simulink model "enfas"  (R2020b)
settings: Solver=VariableStepAuto  StartTime=0.0  StopTime=stop_time  RelTol=tolerance
model workspace (MAT data in the model file):
  R = 40
  a = 220
  freq = 314.16
values from neighbouring files (symbols this model uses):
  amplitude = 220    [lab1.m]
  L = 95 * 10^-3    (= 0.095)    [lab1.m]
settings Model: Creator=axelfroborg  LastModifiedBy=axelfroborg

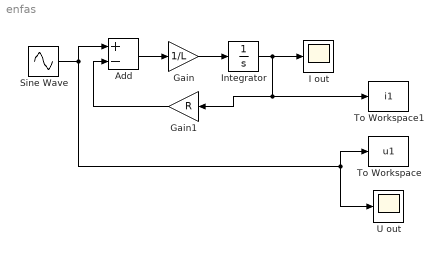
== system enfas ==
  Add : Sum  Inputs=+-
  Gain : Gain  Gain=1/L
  Gain1 : Gain  Gain=R
  I out : Scope
  Integrator : Integrator
  Sine Wave : Sin  Amplitude=amplitude  Frequency=freq  SampleTime=0
  To Workspace : ToWorkspace  VariableName=u1  SampleTime=-1
  To Workspace1 : ToWorkspace  VariableName=i1  SampleTime=-1
  U out : Scope
  wires:
  Integrator/1 -> Gain1/1, To Workspace1/1, I out/1
  Add/1 -> Gain/1
  Gain/1 -> Integrator/1
  Gain1/1 -> Add/2
  Sine Wave/1 -> U out/1, To Workspace/1, Add/1
